simulink model "task2"  (R2024a)
settings: Solver=VariableStepAuto  StartTime=0.0  StopTime=10.0  MaxStep=0.1  RelTol=1e-3
undefined symbols (not defined in the file): A, C, L, x0, x0_hat
settings Model: Creator=sizgr  LastModifiedBy=sizgr

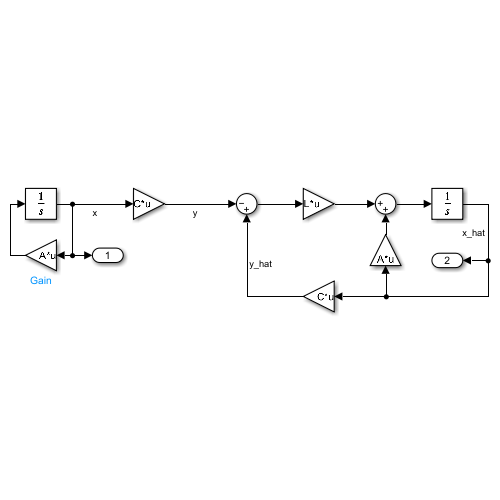
[thumbnail: Simulink's stored preview of the top-level diagram]
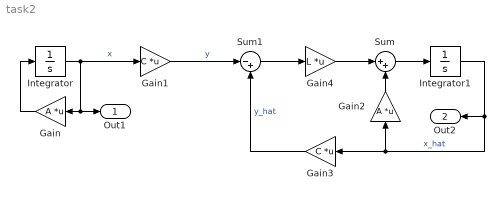
== system task2 ==
  Gain : Gain  Gain=A  Multiplication=Matrix(K*u)
  Gain1 : Gain  Gain=C  Multiplication=Matrix(K*u)
  Gain2 : Gain  Gain=A  Multiplication=Matrix(K*u)
  Gain3 : Gain  Gain=C  Multiplication=Matrix(K*u)
  Gain4 : Gain  Gain=L  Multiplication=Matrix(K*u)
  Integrator : Integrator  InitialCondition=x0
  Integrator1 : Integrator  InitialCondition=x0_hat
  Sum : Sum  Inputs=|++
  Sum1 : Sum  Inputs=|-+
  Out1 : Outport
  Out2 : Outport  Port=2
  wires:
  Integrator/1 -> Out1/1, Gain/1, Gain1/1  "x"
  Gain/1 -> Integrator/1
  Gain1/1 -> Sum1/1  "y"
  Gain2/1 -> Sum/2
  Integrator1/1 -> Out2/1, Gain2/1, Gain3/1  "x_hat"
  Sum/1 -> Integrator1/1
  Gain3/1 -> Sum1/2  "y_hat"
  Sum1/1 -> Gain4/1
  Gain4/1 -> Sum/1
